simulink model "dynamic_model_euler_with_model_base"  (R2021b)
settings: Solver=FixedStepAuto  StartTime=0.0  StopTime=simTime  FixedStep=sim_dt  RelTol=1e-3
undefined symbols (not defined in the file): Angle, Axis, d, g, J_platf, m_mass, m_platf, p, q0, roff, sim_dt, tau, umax, w0
libraries: matrix_library x2, sharedtransform x2, robotcorelib x1, dspindex x1
settings Model: SimulationMode=accelerator  Creator=piszy  LastModifiedBy=krzysztof
settings SolverCC: ZeroCrossControl=DisableAll  AlgebraicLoopSolver=TrustRegion
settings DataIOCC: SaveOutput=off  SaveTime=off
settings OptimizationCC: BlockReduction=off  DefaultParameterBehavior=Inlined  BufferReuse=off
settings ModelReferenceCC: ModelReferenceNumInstancesAllowed=Single
settings SFSimCC: CustomCodeUndefinedFunction=UseInterfaceOnly
settings GRTTargetCC: CombineOutputUpdateFcns=off  MatFileLogging=off

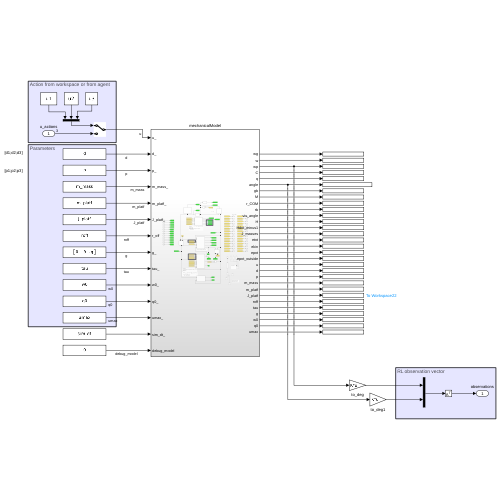
[thumbnail: Simulink's stored preview of the top-level diagram]
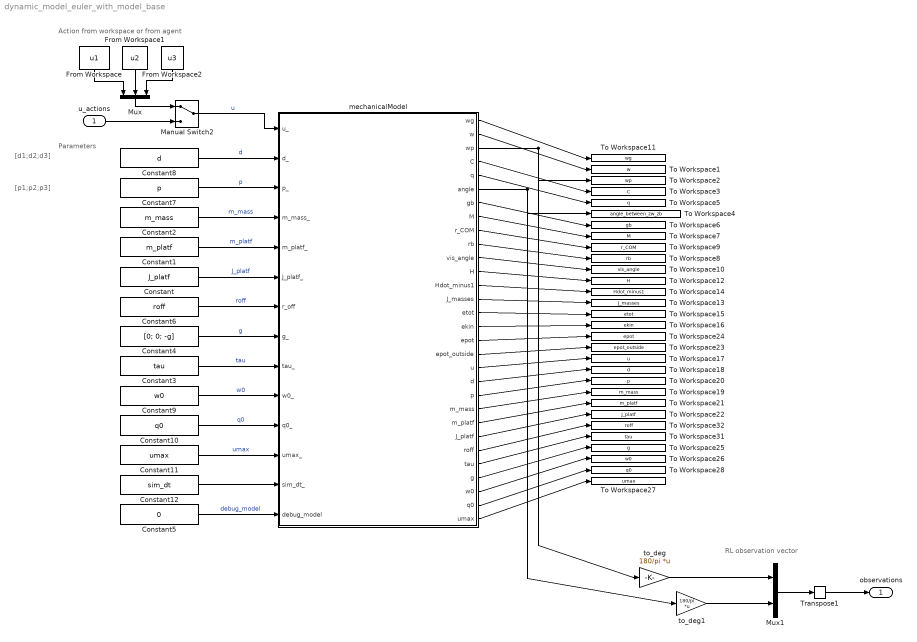
== system dynamic_model_euler_with_model_base ==
  note: Parameters
  note: Action from workspace or from agent
  note: RL observation vector
  note: [p1;p2;p3]
  note: [d1;d2;d3]
  u_actions : Inport  PortDimensions=[3]
  Constant : Constant  Value=J_platf
  Constant1 : Constant  Value=m_platf
  Constant10 : Constant  Value=q0
  Constant11 : Constant  Value=umax
  Constant12 : Constant  Value=sim_dt
  Constant2 : Constant  Value=m_mass
  Constant3 : Constant  Value=tau
  Constant4 : Constant  Value=[0; 0; -g]
  Constant5 : Constant  Value=0
  Constant6 : Constant  Value=roff
  Constant7 : Constant  Value=p
  Constant8 : Constant  Value=d
  Constant9 : Constant  Value=w0
  From Workspace : FromWorkspace  VariableName=u1
  From Workspace1 : FromWorkspace  VariableName=u2
  From Workspace2 : FromWorkspace  VariableName=u3
  Manual Switch2 : ManualSwitch
  Mux : Mux  Inputs=3
  Mux1 : Mux  Inputs=2
  To Workspace1 : ToWorkspace  VariableName=w  SampleTime=-1
  To Workspace10 : ToWorkspace  VariableName=vis_angle  SampleTime=-1
  To Workspace11 : ToWorkspace  VariableName=wg  SampleTime=-1
  To Workspace12 : ToWorkspace  VariableName=H  SampleTime=-1
  To Workspace13 : ToWorkspace  VariableName=J_masses  SampleTime=-1
  To Workspace14 : ToWorkspace  VariableName=Hdot_minus1  SampleTime=-1
  To Workspace15 : ToWorkspace  VariableName=etot  SampleTime=-1
  To Workspace16 : ToWorkspace  VariableName=ekin  SampleTime=-1
  To Workspace17 : ToWorkspace  VariableName=u  SampleTime=-1
  To Workspace18 : ToWorkspace  VariableName=d  SampleTime=-1
  To Workspace19 : ToWorkspace  VariableName=m_mass  SampleTime=-1
  To Workspace2 : ToWorkspace  VariableName=wp  SampleTime=-1
  To Workspace20 : ToWorkspace  VariableName=p  SampleTime=-1
  To Workspace21 : ToWorkspace  VariableName=m_platf  SampleTime=-1
  To Workspace22 : ToWorkspace  VariableName=J_platf  SampleTime=-1
  To Workspace23 : ToWorkspace  VariableName=epot_outside  SampleTime=-1
  To Workspace24 : ToWorkspace  VariableName=epot  SampleTime=-1
  To Workspace25 : ToWorkspace  VariableName=g  SampleTime=-1
  To Workspace26 : ToWorkspace  VariableName=w0  SampleTime=-1
  To Workspace27 : ToWorkspace  VariableName=umax  SampleTime=-1
  To Workspace28 : ToWorkspace  VariableName=q0  SampleTime=-1
  To Workspace3 : ToWorkspace  VariableName=C  SampleTime=-1
  To Workspace31 : ToWorkspace  VariableName=tau  SampleTime=-1
  To Workspace32 : ToWorkspace  VariableName=roff  SampleTime=-1
  To Workspace4 : ToWorkspace  VariableName=angle_between_zw_zb  SampleTime=-1
  To Workspace5 : ToWorkspace  VariableName=q  SampleTime=-1
  To Workspace6 : ToWorkspace  VariableName=gb  SampleTime=-1
  To Workspace7 : ToWorkspace  VariableName=M  SampleTime=-1
  To Workspace8 : ToWorkspace  VariableName=rb  SampleTime=-1
  To Workspace9 : ToWorkspace  VariableName=r_COM  SampleTime=-1
  Transpose1 : matrix_library/Transpose
      settings: SourceProductBaseCode=SL
  mechanicalModel : Subsystem
  to_deg : Gain  Gain=180/pi  Multiplication=Matrix(K*u)
  to_deg1 : Gain  Gain=180/pi  Multiplication=Matrix(K*u)
  observations : Outport
  wires:
  From Workspace/1 -> Mux/1
  From Workspace1/1 -> Mux/2
  From Workspace2/1 -> Mux/3
  Mux/1 -> Manual Switch2/1
  Manual Switch2/1 -> mechanicalModel/1(u_)  "u"
  u_actions/1 -> Manual Switch2/2
  Mux1/1 -> Transpose1/1
  Transpose1/1 -> observations/1
  Constant2/1 -> mechanicalModel/4(m_mass_)  "m_mass"
  Constant5/1 -> mechanicalModel/14(debug_model)  "debug_model"
  Constant8/1 -> mechanicalModel/2(d_)  "d"
  Constant7/1 -> mechanicalModel/3(p_)  "p"
  Constant1/1 -> mechanicalModel/5(m_platf_)  "m_platf"
  Constant3/1 -> mechanicalModel/9(tau_)  "tau"
  Constant6/1 -> mechanicalModel/7(r_off)  "roff"
  Constant4/1 -> mechanicalModel/8(g_)  "g"
  Constant/1 -> mechanicalModel/6(J_platf_)  "J_platf"
  mechanicalModel/6(angle) -> to_deg1/1, To Workspace4/1
  mechanicalModel/3(wp) -> to_deg/1, To Workspace2/1
  to_deg/1 -> Mux1/1
  to_deg1/1 -> Mux1/2
  Constant9/1 -> mechanicalModel/10(w0_)  "w0"
  Constant10/1 -> mechanicalModel/11(q0_)  "q0"
  Constant11/1 -> mechanicalModel/12(umax_)  "umax"
  Constant12/1 -> mechanicalModel/13(sim_dt_)
  mechanicalModel/1(wg) -> To Workspace11/1
  mechanicalModel/2(w) -> To Workspace1/1
  mechanicalModel/4(C) -> To Workspace3/1
  mechanicalModel/5(q) -> To Workspace5/1
  mechanicalModel/7(gb) -> To Workspace6/1
  mechanicalModel/8(M) -> To Workspace7/1
  mechanicalModel/9(r_COM) -> To Workspace9/1
  mechanicalModel/10(rb) -> To Workspace8/1
  mechanicalModel/11(vis_angle) -> To Workspace10/1
  mechanicalModel/12(H) -> To Workspace12/1
  mechanicalModel/13(Hdot_minus1) -> To Workspace14/1
  mechanicalModel/14(J_masses) -> To Workspace13/1
  mechanicalModel/15(etot) -> To Workspace15/1
  mechanicalModel/16(ekin) -> To Workspace16/1
  mechanicalModel/17(epot) -> To Workspace24/1
  mechanicalModel/18(epot_outside) -> To Workspace23/1
  mechanicalModel/19(u) -> To Workspace17/1
  mechanicalModel/20(d) -> To Workspace18/1
  mechanicalModel/21(p) -> To Workspace20/1
  mechanicalModel/22(m_mass) -> To Workspace19/1
  mechanicalModel/23(m_platf) -> To Workspace21/1
  mechanicalModel/24(J_platf) -> To Workspace22/1
  mechanicalModel/25(roff) -> To Workspace32/1
  mechanicalModel/26(tau) -> To Workspace31/1
  mechanicalModel/27(g) -> To Workspace25/1
  mechanicalModel/28(w0) -> To Workspace26/1
  mechanicalModel/29(q0) -> To Workspace28/1
  mechanicalModel/30(umax) -> To Workspace27/1

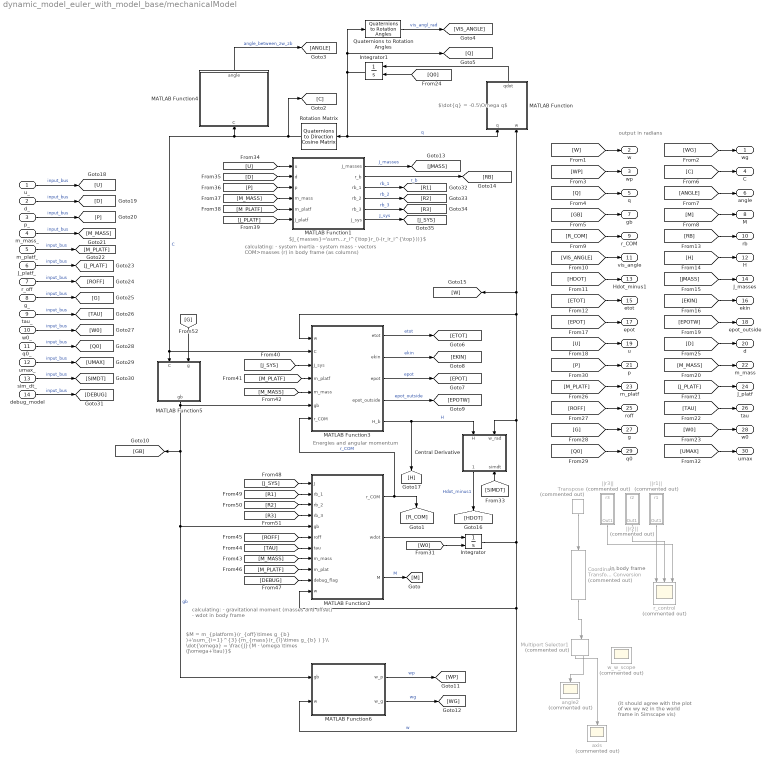
== system dynamic_model_euler_with_model_base/mechanicalModel ==
  note: $J_{masses}=\sum_{i=1}^{3}{m_{i}(I(r_i^{\top}r_i)-(r_ir_i^{\top}))}$
  note: $\dot{q} = -0.5\Omega q$
  note: $M = m_{platform}(r_{off}\times g_{b} )+\sum_{i=1}^{3}{m_{mass}(r_{i}\times g_{b} ) }\\ \dot{\omega} = \frac{J}{M - \omega \times (J\omega+\tau)}$
  note: (it should agree with the plot of wx wy wz in the world frame in Simscape vis)
  note: calculating:
      | - system inertia
      | - system mass
      | - vectors COM>masses (r) in body frame
      | (as columns)
  note: calculating:
      | - gravitational moment (masses and offset)
      | - wdot
      | in body frame
  note: in body frame
  note: Energies and angular momentum
  note: output in radians
  u_ : Inport
  d_ : Inport  Port=2
  p_ : Inport  Port=3
  m_mass_ : Inport  Port=4
  m_platf_ : Inport  Port=5
  J_platf_ : Inport  Port=6
  r_off : Inport  Port=7
  g_ : Inport  Port=8
  tau_ : Inport  Port=9
  w0_ : Inport  Port=10
  q0_ : Inport  Port=11
  umax_ : Inport  Port=12
  sim_dt_ : Inport  Port=13
  debug_model : Inport  Port=14
  Central Derivative : Subsystem
      settings: PortSchema="{\"entries\":[{\"content\":{\"sides\":[{\"content\":{\"connectorIds\":[\"In1\",\"In2\"]},\"type\":\"ConnectorPlacement.EquallySpacedRectSide\",\"uuid\":\"1383cf58-ed2e-4d76-b2bd-bc812874c5c5\"},{\"content\":{\"connectorIds\":[\"Out1\",\"In3\"],\"side\":\"RIGHT\"},\"type\":\"ConnectorPlacement.EquallySpacedRectSide\",\"uuid\":\"b1333be6-c310-4c35-a541-4e98fbac6c75\"},{\"content\":{\"connectorIds\":[],\"side\":\"TOP\"},\"type\":\"ConnectorPlacement.EquallySpacedRectSide\",\"uuid\":\"9de10ece-9fa2-48e9-be23-db895089292f\"}]},\"type\":\"ConnectorPlacement.EquallySpacedConnector\",\"uuid\":\"8dd4b87f-23e7-464d-a0c4-c49a8f880c8a\"}],\"packageUris\":[\"http://schema.mathworks.com/mf0/Connector/R2020b\"],\"version\":\"1.0\"}"
  Coordinate Transformation Conversion : robotcorelib/Coordinate Transformation Conversion  Commented=on  InputRepresentation=Rotation Matrix  InputEulerSequence=ZYX  ShowTrVecInputPort=on  OutputRepresentation=Axis-Angle  OutputEulerSequence=ZYX  ShowTrVecOutputPort=on  SimulateUsing=Interpreted execution
      settings: SourceProductBaseCode=NV,RO,RR,UV
  Integrator : Integrator  InitialConditionSource=external  InitialCondition=w0
  Integrator1 : Integrator  InitialConditionSource=external  InitialCondition=q0
  MATLAB Function : MATLAB Function  TreatAsAtomicUnit=on
  MATLAB Function1 : MATLAB Function  TreatAsAtomicUnit=on
  MATLAB Function2 : MATLAB Function  TreatAsAtomicUnit=on
  MATLAB Function3 : MATLAB Function  TreatAsAtomicUnit=on
  MATLAB Function4 : MATLAB Function  TreatAsAtomicUnit=on
  MATLAB Function5 : MATLAB Function  TreatAsAtomicUnit=on
  MATLAB Function6 : MATLAB Function  TreatAsAtomicUnit=on
  Multiport Selector1 : dspindex/Multiport Selector  Commented=on  rowsOrCols=Rows  idxCellArray={1:3,4}  idxErrMode=Clip Index
  Quaternions to Rotation Angles : sharedtransform/Quaternions to Rotation Angles  rotationOrder=XYZ  aMode=aMode
      settings: SourceProductBaseCode=AE,PW,DR,MT,UV,VE
  Rotation Matrix : sharedtransform/Quaternions to  Direction Cosine Matrix  aMode=aMode
      settings: SourceProductBaseCode=AE,PW,DR,MT,UV,VE
  Transpose : matrix_library/Transpose  Commented=on
      settings: SourceProductBaseCode=SL
  angle2 : Scope  Commented=on
  axis : Scope  Commented=on
  r_control : Scope  Commented=on  NumInputPorts=3
  w_w_scope : Scope  Commented=on
  ||r1|| : Subsystem  Commented=on
  ||r2|| : Subsystem  Commented=on
  ||r3|| : Subsystem  Commented=on
  wg : Outport
  w : Outport  Port=2
  wp : Outport  Port=3
  C : Outport  Port=4
  q : Outport  Port=5
  angle : Outport  Port=6
  gb : Outport  Port=7
  M : Outport  Port=8
  r_COM : Outport  Port=9
  rb : Outport  Port=10
  vis_angle : Outport  Port=11
  H : Outport  Port=12
  Hdot_minus1 : Outport  Port=13
  J_masses : Outport  Port=14
  etot : Outport  Port=15
  ekin : Outport  Port=16
  epot : Outport  Port=17
  epot_outside : Outport  Port=18
  u : Outport  Port=19
  d : Outport  Port=20
  p : Outport  Port=21
  m_mass : Outport  Port=22
  m_platf : Outport  Port=23
  J_platf : Outport  Port=24
  roff : Outport  Port=25
  tau : Outport  Port=26
  g : Outport  Port=27
  w0 : Outport  Port=28
  q0 : Outport  Port=29
  umax : Outport  Port=30
  wires:
  Integrator1/1 -> MATLAB Function/1(q), Rotation Matrix/1, [Q], Quaternions to Rotation Angles/1  "q"
  MATLAB Function/1(qdot) -> Integrator1/1
  Transpose/1 -> Coordinate Transformation Conversion/1
  Coordinate Transformation Conversion/1 -> Multiport Selector1/1
  Multiport Selector1/2 -> angle2/1
  Multiport Selector1/1 -> axis/1
  ||r3||/1(Out1) -> r_control/3
  ||r1||/1(Out1) -> r_control/1
  ||r2||/1(Out1) -> r_control/2
  [G] -> MATLAB Function5/2(g)
  MATLAB Function2/2(wdot) -> Integrator/1
  Integrator/1 -> MATLAB Function6/2(w), MATLAB Function2/11(w), MATLAB Function3/1(w), MATLAB Function/2(w), [W], Central Derivative/2(w_rad)  "w"
  MATLAB Function5/1(gb) -> MATLAB Function3/6(gb), MATLAB Function6/1(gb), MATLAB Function2/5(gb), [GB]  "gb"
  MATLAB Function2/3(M) -> [M]  "M"
  MATLAB Function3/2(ekin) -> [EKIN]  "ekin"
  MATLAB Function3/3(epot) -> [EPOT]  "epot"
  MATLAB Function3/1(etot) -> [ETOT]  "etot"
  MATLAB Function6/1(w_p) -> [WP]  "wp"
  MATLAB Function6/2(w_g) -> [WG]  "wg"
  MATLAB Function1/1(J_masses) -> [JMASS]  "J_masses"
  MATLAB Function2/1(r_COM) -> [R_COM], MATLAB Function3/7(r_COM)  "r_COM"
  MATLAB Function3/4(epot_outside) -> [EPOTW]  "epot_outside"
  Rotation Matrix/1 -> [C], MATLAB Function3/2(C), MATLAB Function5/1(C), MATLAB Function4/1(C)  "C"
  MATLAB Function1/2(r_b) -> [RB]  "r_b"
  MATLAB Function4/1(angle) -> [ANGLE]  "angle_between_zw_zb"
  Quaternions to Rotation Angles/1 -> [VIS_ANGLE]  "vis_angl_rad"
  [Q0] -> Integrator1/2
  [W0] -> Integrator/2
  MATLAB Function3/5(H_b) -> Central Derivative/1(H), [H]  "H"
  Central Derivative/1(Hdot_minus1) -> [HDOT]  "Hdot_minus1"
  [SIMDT] -> Central Derivative/3(simdt)
  [UMAX] -> umax/1
  [W] -> w/1
  [WP] -> wp/1
  [Q] -> q/1
  [GB] -> gb/1
  [R_COM] -> r_COM/1
  [VIS_ANGLE] -> vis_angle/1
  [HDOT] -> Hdot_minus1/1
  [ETOT] -> etot/1
  [EPOT] -> epot/1
  [U] -> u/1
  [P] -> p/1
  [M_PLATF] -> m_platf/1
  [ROFF] -> roff/1
  [G] -> g/1
  [Q0] -> q0/1
  [W0] -> w0/1
  [TAU] -> tau/1
  [J_PLATF] -> J_platf/1
  [M_MASS] -> m_mass/1
  [D] -> d/1
  [EPOTW] -> epot_outside/1
  [EKIN] -> ekin/1
  [JMASS] -> J_masses/1
  [H] -> H/1
  [RB] -> rb/1
  [M] -> M/1
  [ANGLE] -> angle/1
  [C] -> C/1
  [WG] -> wg/1
  umax_/1 -> [UMAX]  "input_bus"
  sim_dt_/1 -> [SIMDT]  "input_bus"
  q0_/1 -> [Q0]  "input_bus"
  w0_/1 -> [W0]  "input_bus"
  tau_/1 -> [TAU]  "input_bus"
  g_/1 -> [G]  "input_bus"
  r_off/1 -> [ROFF]  "input_bus"
  J_platf_/1 -> [J_PLATF]  "input_bus"
  m_platf_/1 -> [M_PLATF]  "input_bus"
  m_mass_/1 -> [M_MASS]  "input_bus"
  p_/1 -> [P]  "input_bus"
  d_/1 -> [D]  "input_bus"
  u_/1 -> [U]  "input_bus"
  debug_model/1 -> [DEBUG]  "input_bus"
  [U] -> MATLAB Function1/1(u)
  [D] -> MATLAB Function1/2(d)
  [P] -> MATLAB Function1/3(p)
  [M_MASS] -> MATLAB Function1/4(m_mass)
  [M_PLATF] -> MATLAB Function1/5(m_platf)
  [J_PLATF] -> MATLAB Function1/6(J_platf)
  MATLAB Function1/3(rb_1) -> [R1]  "rb_1"
  MATLAB Function1/4(rb_2) -> [R2]  "rb_2"
  MATLAB Function1/5(rb_3) -> [R3]  "rb_3"
  MATLAB Function1/6(J_sys) -> [J_SYS]  "J_sys"
  [J_SYS] -> MATLAB Function3/3(J_sys)
  [M_MASS] -> MATLAB Function3/5(m_mass)
  [M_PLATF] -> MATLAB Function3/4(m_platf)
  [M_MASS] -> MATLAB Function2/8(m_mass)
  [TAU] -> MATLAB Function2/7(tau)
  [ROFF] -> MATLAB Function2/6(roff)
  [M_PLATF] -> MATLAB Function2/9(m_plat)
  [DEBUG] -> MATLAB Function2/10(debug_flag)
  [J_SYS] -> MATLAB Function2/1(J)
  [R1] -> MATLAB Function2/2(rb_1)
  [R2] -> MATLAB Function2/3(rb_2)
  [R3] -> MATLAB Function2/4(rb_3)

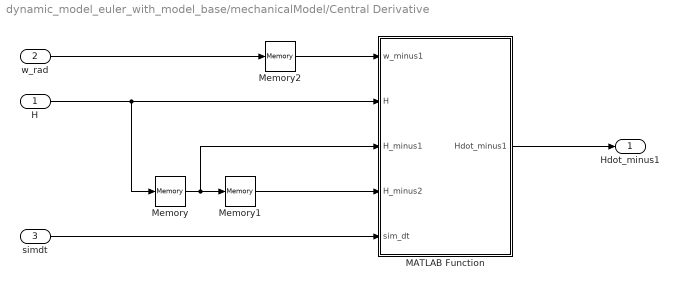
== system dynamic_model_euler_with_model_base/mechanicalModel/Central Derivative ==
  H : Inport
  w_rad : Inport  Port=2
  simdt : Inport  Port=3
  MATLAB Function : MATLAB Function  TreatAsAtomicUnit=on
  Memory : Memory
  Memory1 : Memory
  Memory2 : Memory
  Hdot_minus1 : Outport
  wires:
  Memory1/1 -> MATLAB Function/4(H_minus2)
  H/1 -> MATLAB Function/2(H), Memory/1
  Memory2/1 -> MATLAB Function/1(w_minus1)
  simdt/1 -> MATLAB Function/5(sim_dt)
  Memory/1 -> MATLAB Function/3(H_minus1), Memory1/1
  MATLAB Function/1(Hdot_minus1) -> Hdot_minus1/1
  w_rad/1 -> Memory2/1

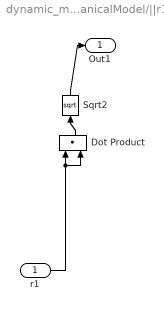
== system dynamic_model_euler_with_model_base/mechanicalModel/||r1|| ==
  r1 : Inport
  Dot Product : DotProduct  RndMeth=Nearest  InputSameDT=on  OutDataTypeStr=Inherit: Inherit via internal rule
  Sqrt2 : Sqrt  SaturateOnIntegerOverflow=on
  Out1 : Outport
  wires:
  Dot Product/1 -> Sqrt2/1
  r1/1 -> Dot Product/2, Dot Product/1
  Sqrt2/1 -> Out1/1

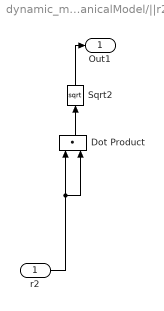
== system dynamic_model_euler_with_model_base/mechanicalModel/||r2|| ==
  r2 : Inport
  Dot Product : DotProduct  RndMeth=Nearest  InputSameDT=on  OutDataTypeStr=Inherit: Inherit via internal rule
  Sqrt2 : Sqrt  SaturateOnIntegerOverflow=on
  Out1 : Outport
  wires:
  Dot Product/1 -> Sqrt2/1
  r2/1 -> Dot Product/1, Dot Product/2
  Sqrt2/1 -> Out1/1

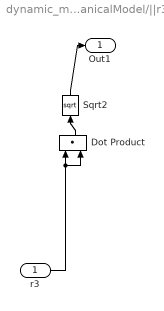
== system dynamic_model_euler_with_model_base/mechanicalModel/||r3|| ==
  r3 : Inport
  Dot Product : DotProduct  RndMeth=Nearest  InputSameDT=on  OutDataTypeStr=Inherit: Inherit via internal rule
  Sqrt2 : Sqrt  SaturateOnIntegerOverflow=on
  Out1 : Outport
  wires:
  Dot Product/1 -> Sqrt2/1
  r3/1 -> Dot Product/2, Dot Product/1
  Sqrt2/1 -> Out1/1

== matlab function dynamic_model_euler_with_model_base/mechanicalModel/Central Derivative/MATLAB Function ==
  data: w_minus1 input; H input; H_minus1 input; Hdot_minus1 output; H_minus2 input; sim_dt input
function Hdot_minus1 = fcn(w_minus1,H,H_minus1,H_minus2, sim_dt)
   H_in_body_dot_minus1 = (H - H_minus2)/2/sim_dt;
   Hdot_minus1 = H_in_body_dot_minus1 + cross(w_minus1,H_minus1);

== matlab function dynamic_model_euler_with_model_base/mechanicalModel/MATLAB Function5 ==
  data: C input; gb output; g input
function gb = gbodyframe(C,g)
gb = C*g;

== matlab function dynamic_model_euler_with_model_base/mechanicalModel/MATLAB Function3 ==
  data: w input; C input; J_sys input; m_platf input; m_mass input; gb input; etot output; ekin output; epot output; epot_outside output; H_b output; r_COM input
function [etot,ekin,epot,epot_outside, H_b] = fcn(w,C,J_sys, m_platf,m_mass,gb,r_COM)
% J_sys = concat_in(:,1:3);
% rb1 = concat_in(:,6);
% rb2 = concat_in(:,5);
% rb3 = concat_in(:,4);

% disp(r_COM)

ekin = 0.5*(w)'*J_sys*(w);

epot = (3*m_mass + m_platf) * gb(3) * vecnorm(r_COM);
%epot = m_platf*gb(3)*vecnorm(r_COM);

r_COM_w = C'*r_COM;
epot_outside = (3*m_mass + m_platf) * vecnorm(gb) * r_COM_w(3);

etot = epot+ekin;
%hmag = vecnorm(J*w);

% H_b = [J_sys(1,1)*w(1)-J_sys(1,2)*w(2)-J_sys(1,3)*w(3); 
%     -J_sys(2,1)*w(1)+J_sys(2,2)*w(2)-J_sys(2,3)*w(3); 
%     -J_sys(3,1)*w(1)-J_sys(3,2)*w(2)+J_sys(3,3)*w(3); 
%     ];

H_b = J_sys * w;

== matlab function dynamic_model_euler_with_model_base/mechanicalModel/MATLAB Function ==
  data: q input; w input; qdot output
function qdot = derq(q,w)

w_x = w(1); w_y = w(2); w_z = w(3);

% omega = [ 0     w_z   -w_y    w_x;... 
%           -w_z   0       w_x    w_y;... 
%           w_y   -w_x    0       w_z;... 
%           -w_x   -w_y    -w_z     0];

omega = [ 0      w_x   w_y    w_z;... 
          -w_x   0    -w_z    w_y;... 
          -w_y   w_z    0    -w_x;... 
          -w_z  -w_y   w_x     0];

qdot = -0.5*omega*q;

== matlab function dynamic_model_euler_with_model_base/mechanicalModel/MATLAB Function2 ==
  data: r_COM output; J input; rb_1 input; rb_2 input; rb_3 input; gb input; roff input; tau input; m_mass input; m_plat input; debug_flag input; w input; wdot output; M output
function [r_COM, wdot, M] = fcn(J, rb_1, rb_2, rb_3, gb, roff, tau, m_mass, m_plat, debug_flag,w)

% concatenated along columns
% J = concat_in(:,1:3);
% rb_1 = concat_in(:,6);
% rb_2 = concat_in(:,5);
% rb_3 = concat_in(:,4);
if debug_flag
    disp("Inside gravitational torque and wdot calculation function:")
    disp("J"),disp(J)
    disp("rb1"),disp(rb_1)
    disp("rb2"),disp(rb_2)
    disp("rb3"),disp(rb_3)
    disp("gb"),disp(gb)
    disp("roff"),disp(roff)
    disp("tau"),disp(tau)
    disp("w"),disp(w)
end

r_COM = (m_mass*rb_1 + m_mass*rb_2 + m_mass*rb_3 + m_plat*roff)/(3*m_mass+m_plat);

%M = m_plat*cross(roff,gb) + m_mass*cross(rb_1,gb) + m_mass*cross(rb_2,gb) + m_mass*cross(rb_3,gb);
M = (3*m_mass+m_plat)*cross(r_COM,gb);

wdot = J\(M-cross(w,(J*w))+tau); %given that dt(Jw)/dt = J * dw/dt

== matlab function dynamic_model_euler_with_model_base/mechanicalModel/MATLAB Function1 ==
  data: J_masses output; r_b output; rb_1 output; rb_2 output; rb_3 output; J_sys output; u input; d input; p input; m_mass input; m_platf input; J_platf input
function [J_masses, r_b, rb_1, rb_2, rb_3,  J_sys] = fcn(u, d, p, m_mass, m_platf, J_platf)
% [r1x r1y r1z; r2x r2y r2z; r3x r3y r3z]
% [p1x p1y p1z; p2x p2y p2z; p3x p3y p3z]
% [	d1x d1y d1z; 
% 	d2x d2y d2z; 
% 	d3x d3y d3z]
% [u1; u2; u3] !!!!==== jestem przekonany, że to kolumna
% r = p + u/||d||*d
% r is a sum of the p vector and a vector of length u that is along
% d vector

% d' = 	[d1x d2x d3x; 
%		 d1y d2y d3y; 
%		 d1z d2z d3z]
% vecnorm(d') = 	[||d1|| ||d2|| ||d3||]
% (vecnorm(d'))' = 	[||d1||;||d2||;||d3||]
% (u ./ (vecnorm(d'))') = [u1/||d1||; u2/||d2||; u3/||d3||]
% (u ./ (vecnorm(d'))') .* d = [	u1/||d1||*d1x	u1/||d1||*d1y u1/||d1||*d1z;
%								    u2/||d2||*d2x	u2/||d2||*d2y u2/||d2||*d2z;
%								    u3/||d3||*d3x	u3/||d3||*d3y u3/||d3||*d3z;
r_b = p + (u ./ (vecnorm(d'))') .* d;

% make rb column vectors
rb_1 = r_b(1,:)'; rb_2 = r_b(2,:)'; rb_3 = r_b(3,:)'; 

J_masses =    m_mass*(eye(3)*(rb_1' * rb_1) - rb_1 * rb_1')...
            + m_mass*(eye(3)*(rb_2' * rb_2) - rb_2 * rb_2')... 
            + m_mass*(eye(3)*(rb_3' * rb_3) - rb_3 * rb_3');

% to Eq. 6 in (Zagórski 2020)

J_sys = J_masses + J_platf;
% m_sys = m_platf + 3 * m_mass;

== matlab function dynamic_model_euler_with_model_base/mechanicalModel/MATLAB Function4 ==
  data: C input; angle output
function angle    = calculate_constraint(C)
%     rw1 = Q'*r1;
%     rw2 = Q'*r2;
%     rw3 = Q'*r3;
%     w_w = Q'*w;
    % k_prim - coordinates of body frame versor in the inertial frame
    k_prim = C' * [0; 0; 1];
    % angle = acos( round( dot( k_prim, [0; 0; 1]) * 1e13) / 1e13); 
    angle = acos ( round( k_prim(3) * 1e13 ) / 1e13);
    % beacuse [0; 0; 1] => k_prim_x*0 and k_prim_y*0
    % and ||k||||k'|| = 1
    % rounding to 13 decimal places to get rid of the situation that cos due to calculation error > 1
end

== matlab function dynamic_model_euler_with_model_base/mechanicalModel/MATLAB Function6 ==
  data: gb input; w input; w_p output; w_g output
function [w_p, w_g] = projection_operator(gb,w)
operator =  eye - (gb * gb')/((vecnorm(gb))^2);
w_p = (operator * w);
w_g = (w - w_p);
